simulink model "Stirred_tank_heater_PIC_Xilinx"  (R2017b)
settings: Solver=VariableStepAuto  StartTime=0.0  StopTime=4  RelTol=1e-3
libraries: xbsIndex_r4 x10
settings Model: Creator=HP  LastModifiedBy=HP

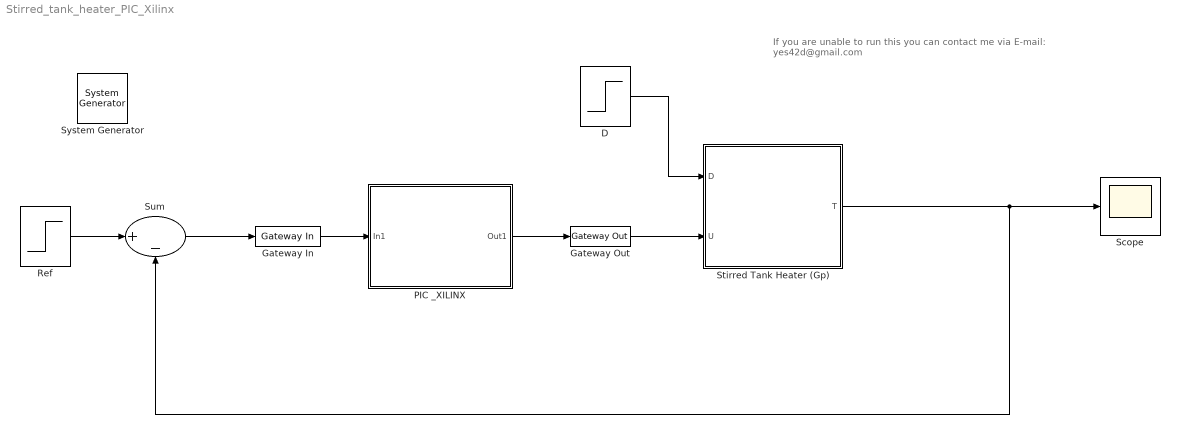
== system Stirred_tank_heater_PIC_Xilinx ==
  note: If you are unable to run this you can contact me
      | via E-mail: yes42d@gmail.com
  " System Generator" : xbsIndex_r4/ System Generator  Tag=genX  xilinxfamily=kintex7  part=xc7k325t  speed=-3  package=fbg676  synthesis_tool=Vivado  clock_wrapper=Clock Enables  directory=./netlist  proj_type=Vivado  Synth_file=Vivado Synthesis Defaults  Impl_file=Vivado Implementation Defaults  testbench=off  simulink_period=1/10e4  sysclk_period=10  dcm_input_clock_period=10  incr_netlist=off  trim_vbits=Everywhere in SubSystem  dbl_ovrd=According to Block Masks  core_generation=According to Block Masks  run_coregen=off  deprecated_control=off  eval_field=0  block_type=sysgen
  D : Step  Time=2  After=0  SampleTime=0.01
  Gateway In : xbsIndex_r4/Gateway In  gui_display_data_type=Floating-point  arith_type=Floating-point  n_bits=16  bin_pt=14  preci_type=Double  exp_width=8  frac_width=24  rows=1  columns=1  quantization="Round  (unbiased: +/- Inf)"  overflow=Saturate  period=1/10e4  UseAsADC=off  ADCChannel='1'  interface=None  automatic_assignment=on  address_offset=hex2dec('00')  intf_name=''  intf_description=''  default_value=0  timing_constraint=None  locs_specified=off  LOCs={}  io_standard={}  inherit_from_input=off  hdl_port=on  dbl_ovrd=off  block_type=gatewayin
  Gateway Out : xbsIndex_r4/Gateway Out  inherit_from_input=off  hdl_port=on  rows=1  columns=1  UseAsDAC=off  DACChannel='1'  interface=None  automatic_assignment=on  address_offset=hex2dec('00')  intf_name=''  intf_description=''  timing_constraint=None  locs_specified=off  LOCs={}  io_standard={}  block_type=gatewayout
  PIC _XILINX : Subsystem
  Ref : Step  Time=0  SampleTime=0.01
  Scope : Scope
  Stirred Tank Heater (Gp) : Subsystem
  Sum : Sum  Inputs=|+-
  wires:
  PIC _XILINX/1(Out1) -> Gateway Out/1
  Sum/1 -> Gateway In/1
  Gateway In/1 -> PIC _XILINX/1(In1)
  Stirred Tank Heater (Gp)/1(T) -> Sum/2, Scope/1
  Ref/1 -> Sum/1
  D/1 -> Stirred Tank Heater (Gp)/1(D)
  Gateway Out/1 -> Stirred Tank Heater (Gp)/2(U)

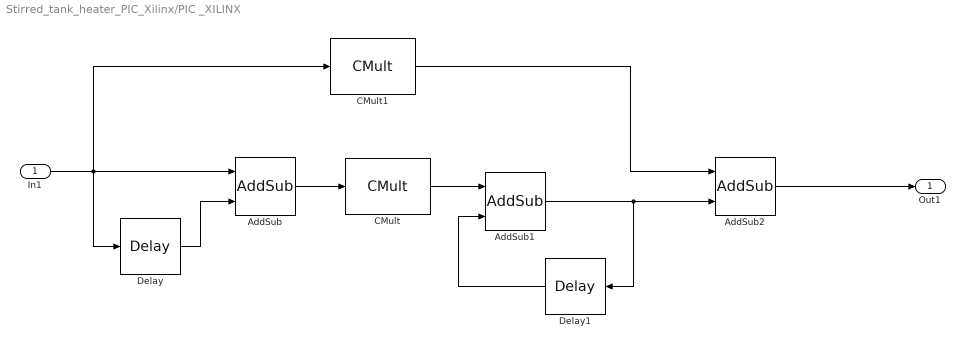
== system Stirred_tank_heater_PIC_Xilinx/PIC _XILINX ==
  In1 : Inport
  AddSub : xbsIndex_r4/AddSub  mode=Addition  use_carryin=off  use_carryout=off  en=off  latency=0  precision=Full  arith_type=Unsigned  n_bits=16  bin_pt=14  quantization=Truncate  overflow=Wrap  use_behavioral_HDL=off  hw_selection=Fabric  pipelined=off  dbl_ovrd=off  block_type=addsub
  AddSub1 : xbsIndex_r4/AddSub  mode=Addition  use_carryin=off  use_carryout=off  en=off  latency=0  precision=Full  arith_type=Unsigned  n_bits=16  bin_pt=14  quantization=Truncate  overflow=Wrap  use_behavioral_HDL=off  hw_selection=Fabric  pipelined=off  dbl_ovrd=off  block_type=addsub
  AddSub2 : xbsIndex_r4/AddSub  mode=Addition  use_carryin=off  use_carryout=off  en=off  latency=0  precision=Full  arith_type=Unsigned  n_bits=16  bin_pt=14  quantization=Truncate  overflow=Wrap  use_behavioral_HDL=off  hw_selection=Fabric  pipelined=off  dbl_ovrd=off  block_type=addsub
  CMult : xbsIndex_r4/CMult  const=36/(2*10e4)  gui_display_data_type=Floating-point  const_n_bits=32  const_bin_pt=28  float_type=Double  exp_bits=8  fraction_bits=24  en=off  latency=0  precision=Full  arith_type="Signed  (2's comp)"  n_bits=16  bin_pt=14  quantization=Truncate  overflow=Wrap  use_behavioral_HDL=off  mem_type=Distributed RAM  pipeline=off  dbl_ovrd=off  block_type=cmult
  CMult1 : xbsIndex_r4/CMult  const=3  gui_display_data_type=Floating-point  const_n_bits=16  const_bin_pt=14  float_type=Double  exp_bits=8  fraction_bits=24  en=off  latency=0  precision=Full  arith_type="Signed  (2's comp)"  n_bits=16  bin_pt=14  quantization=Truncate  overflow=Wrap  use_behavioral_HDL=off  mem_type=Distributed RAM  pipeline=off  dbl_ovrd=off  block_type=cmult
  Delay : xbsIndex_r4/Delay  rst=off  infoeditControl=Selection of Reset will increase slice count due to use of real FFs and instead of SRLs  en=off  latency=1  reg_retiming=off  dbl_ovrd=off  block_type=delay
  Delay1 : xbsIndex_r4/Delay  rst=off  infoeditControl=Selection of Reset will increase slice count due to use of real FFs and instead of SRLs  en=off  latency=1  reg_retiming=off  dbl_ovrd=off  block_type=delay
  Out1 : Outport
  wires:
  AddSub1/1 -> AddSub2/2, Delay1/1
  In1/1 -> CMult1/1, AddSub/1, Delay/1
  Delay/1 -> AddSub/2
  AddSub/1 -> CMult/1
  CMult/1 -> AddSub1/1
  Delay1/1 -> AddSub1/2
  AddSub2/1 -> Out1/1
  CMult1/1 -> AddSub2/1

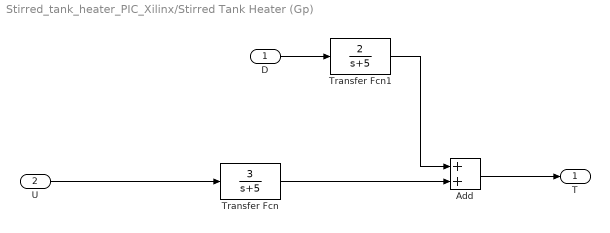
== system Stirred_tank_heater_PIC_Xilinx/Stirred Tank Heater (Gp) ==
  D : Inport
  U : Inport  Port=2
  Add : Sum
  Transfer Fcn : TransferFcn  Numerator=[3]  Denominator=[1 5]
  Transfer Fcn1 : TransferFcn  Numerator=[2]  Denominator=[1 5]
  T : Outport
  wires:
  U/1 -> Transfer Fcn/1
  Add/1 -> T/1
  Transfer Fcn/1 -> Add/2
  Transfer Fcn1/1 -> Add/1
  D/1 -> Transfer Fcn1/1
